simulink library "inp"  (R2021b)
settings: Solver=VariableStepAuto  StartTime=0.0  StopTime=10.0  RelTol=1e-3
undefined symbols (not defined in the file): C_TASK_5MS_S, FALSE, KINP_AcoreReadyToSlp_flg_ovrdflg, KINP_AcoreReadyToSlp_flg_ovrdval, KINP_AllowMovThd_OTA_enum_ovrdflg, KINP_AllowMovThd_OTA_enum_ovrdval, KINP_APSAngleTarget_Deg_ovrdflg, KINP_APSAngleTarget_Deg_ovrdval, KINP_APSDecReq_mps2_ovrdflg, KINP_APSDecReq_mps2_ovrdval, KINP_APSDecReqA_flg_ovrdflg, KINP_APSDecReqA_flg_ovrdval, KINP_APSDFLL_cm_ovrdflg, KINP_APSDFLL_cm_ovrdval, KINP_APSDFLR_cm_ovrdflg, KINP_APSDFLR_cm_ovrdval, KINP_APSDRLL_cm_ovrdflg, KINP_APSDRLL_cm_ovrdval, KINP_APSDRLR_cm_ovrdflg, KINP_APSDRLR_cm_ovrdval, KINP_APSExitCondition_enum_ovrdflg, KINP_APSExitCondition_enum_ovrdval, KINP_APSHWVer_enum_ovrdflg, KINP_APSHWVer_enum_ovrdval, KINP_APSProgressPCT_pct_ovrdflg, KINP_APSProgressPCT_pct_ovrdval, KINP_APSReq_enum_ovrdflg, KINP_APSReq_enum_ovrdval, KINP_APSRQDisplay_enum_ovrdflg, KINP_APSRQDisplay_enum_ovrdval, KINP_APSRqEPASCtrl_flg_ovrdflg, KINP_APSRqEPASCtrl_flg_ovrdval, KINP_APSShiftPosnReq_enum_ovrdval, KINP_APSShiftPosnReq_enum_ovrflg, KINP_APSSpeedCMD_kph_ovrdval, KINP_APSSpeedCMD_kph_ovrflg, KINP_APSStaSystem_enum_ovrdflg, KINP_APSStaSystem_enum_ovrdval, KINP_APSSWVer_enum_ovrdflg, KINP_APSSWVer_enum_ovrdval, KINP_APSVMCReqA_flg_ovrdval, KINP_APSVMCReqA_flg_ovrflg, KINP_APSVRqEPASCtrl_flg_ovrdflg, KINP_APSVRqEPASCtrl_flg_ovrdval, KINP_AuxBattVolmV_mV_ovrdflg, KINP_AuxBattVolmV_mV_ovrdval, KINP_CAASSta_enum_ovrdflg, KINP_CAASSta_enum_ovrdval, KINP_CAASVMCReqA_flg_ovrdval, KINP_CAASVMCReqA_flg_ovrflg, KINP_Chime_enum_ovrdflg, KINP_Chime_enum_ovrdval, KINP_ClearDTCcmd_flg_ovrdflg, KINP_ClearDTCcmd_flg_ovrdval, KINP_EvccAplusPwrUpReq_flg_ovrdflg, KINP_EvccAplusPwrUpReq_flg_ovrdval, KINP_LFID_raw_ovrdval, KINP_LFID_raw_ovrflg, KINP_LRID_raw_ovrdval, KINP_MemOffsetAccX_raw16_ovrdflg ... (+118)
libraries: FVT_lib x595, hcu_lib x1
(part 27 of 27)

== system inp/INP/CAN5/SignalCheck/TBOX1 ==
  BHAL_outputs : Inport
  inp_CanValid_bus : Inport  Port=2
  PowerOffTSet : FVT_lib/inp/can_signal_template  SystemSampleTime=-1  VariantActivationTime=update diagram  Latency=0  AutoFrameSizeCalculation=off
      link override defval: Value=KINP_PowerOffTSet_cnt_defval
      link override fftdec: Value=KINP_PowerOffTSet_cnt_fftdec
      link override fftinc: Value=KINP_PowerOffTSet_cnt_fftinc
      link override fftlim: Value=KINP_PowerOffTSet_cnt_fftlim
      link override invalid: Value=KINP_PowerOffTSet_cnt_invalid
      link override ovrdflg: Value=KINP_PowerOffTSet_cnt_ovrdflg
      link override ovrdval: Value=KINP_PowerOffTSet_cnt_ovrdval
      link override setvalid: Value=KINP_PowerOffTSet_cnt_setvalid
      link override srvcflg: Value=KINP_PowerOffTSet_cnt_srvcflg
      link override srvcval: Value=KINP_PowerOffTSet_cnt_srvcval
  ReDoorLock : FVT_lib/inp/can_signal_template  SystemSampleTime=-1  VariantActivationTime=update diagram  Latency=0  AutoFrameSizeCalculation=off
      link override defval: Value=KINP_ReDoorLock_enum_defval
      link override fftdec: Value=KINP_ReDoorLock_enum_fftdec
      link override fftinc: Value=KINP_ReDoorLock_enum_fftinc
      link override fftlim: Value=KINP_ReDoorLock_enum_fftlim
      link override invalid: Value=KINP_ReDoorLock_enum_invalid
      link override ovrdflg: Value=KINP_ReDoorLock_enum_ovrdflg
      link override ovrdval: Value=KINP_ReDoorLock_enum_ovrdval
      link override setvalid: Value=KINP_ReDoorLock_enum_setvalid
      link override srvcflg: Value=KINP_ReDoorLock_enum_srvcflg
      link override srvcval: Value=KINP_ReDoorLock_enum_srvcval
  ReOutsideMirror : FVT_lib/inp/can_signal_template  SystemSampleTime=-1  VariantActivationTime=update diagram  Latency=0  AutoFrameSizeCalculation=off
      link override defval: Value=KINP_ReOutsideMirror_enum_defval
      link override fftdec: Value=KINP_ReOutsideMirror_enum_fftdec
      link override fftinc: Value=KINP_ReOutsideMirror_enum_fftinc
      link override fftlim: Value=KINP_ReOutsideMirror_enum_fftlim
      link override invalid: Value=KINP_ReOutsideMirror_enum_invalid
      link override ovrdflg: Value=KINP_ReOutsideMirror_enum_ovrdflg
      link override ovrdval: Value=KINP_ReOutsideMirror_enum_ovrdval
      link override setvalid: Value=KINP_ReOutsideMirror_enum_setvalid
      link override srvcflg: Value=KINP_ReOutsideMirror_enum_srvcflg
      link override srvcval: Value=KINP_ReOutsideMirror_enum_srvcval
  RePwrReqTbox : FVT_lib/inp/can_signal_template  SystemSampleTime=-1  VariantActivationTime=update diagram  Latency=0  AutoFrameSizeCalculation=off
      link override defval: Value=KINP_RePwrReqTbox_enum_defval
      link override fftdec: Value=KINP_RePwrReqTbox_enum_fftdec
      link override fftinc: Value=KINP_RePwrReqTbox_enum_fftinc
      link override fftlim: Value=KINP_RePwrReqTbox_enum_fftlim
      link override invalid: Value=KINP_RePwrReqTbox_enum_invalid
      link override ovrdflg: Value=KINP_RePwrReqTbox_enum_ovrdflg
      link override ovrdval: Value=KINP_RePwrReqTbox_enum_ovrdval
      link override setvalid: Value=KINP_RePwrReqTbox_enum_setvalid
      link override srvcflg: Value=KINP_RePwrReqTbox_enum_srvcflg
      link override srvcval: Value=KINP_RePwrReqTbox_enum_srvcval
  RemoteACTemp : FVT_lib/inp/can_signal_template  SystemSampleTime=-1  VariantActivationTime=update diagram  Latency=0  AutoFrameSizeCalculation=off
      link override defval: Value=KINP_RemoteACTemp_C_defval
      link override fftdec: Value=KINP_RemoteACTemp_C_fftdec
      link override fftinc: Value=KINP_RemoteACTemp_C_fftinc
      link override fftlim: Value=KINP_RemoteACTemp_C_fftlim
      link override invalid: Value=KINP_RemoteACTemp_C_invalid
      link override ovrdflg: Value=KINP_RemoteACTemp_C_ovrdflg
      link override ovrdval: Value=KINP_RemoteACTemp_C_ovrdval
      link override setvalid: Value=KINP_RemoteACTemp_C_setvalid
      link override srvcflg: Value=KINP_RemoteACTemp_C_srvcflg
      link override srvcval: Value=KINP_RemoteACTemp_C_srvcval
  RemoteAutoReq : FVT_lib/inp/can_signal_template  SystemSampleTime=-1  VariantActivationTime=update diagram  Latency=0  AutoFrameSizeCalculation=off
      link override defval: Value=KINP_RemoteAutoReq_flg_defval
      link override fftdec: Value=KINP_RemoteAutoReq_flg_fftdec
      link override fftinc: Value=KINP_RemoteAutoReq_flg_fftinc
      link override fftlim: Value=KINP_RemoteAutoReq_flg_fftlim
      link override invalid: Value=KINP_RemoteAutoReq_flg_invalid
      link override ovrdflg: Value=KINP_RemoteAutoReq_flg_ovrdflg
      link override ovrdval: Value=KINP_RemoteAutoReq_flg_ovrdval
      link override setvalid: Value=KINP_RemoteAutoReq_flg_setvalid
      link override srvcflg: Value=KINP_RemoteAutoReq_flg_srvcflg
      link override srvcval: Value=KINP_RemoteAutoReq_flg_srvcval
  Terminator_{1..6} (6 alike) : Terminator
  True_VHAL_PowerOffTSet_cnt : Constant  Value=TRUE  OutDataTypeStr=boolean
  True_VHAL_ReDoorLock_enum : Constant  Value=TRUE  OutDataTypeStr=boolean
  True_VHAL_ReOutsideMirror_enum : Constant  Value=TRUE  OutDataTypeStr=boolean
  True_VHAL_RePwrReqTbox_enum : Constant  Value=TRUE  OutDataTypeStr=boolean
  True_VHAL_RemoteACTemp_C : Constant  Value=TRUE  OutDataTypeStr=boolean
  True_VHAL_RemoteAutoReq_flg : Constant  Value=TRUE  OutDataTypeStr=boolean
  slr1_{1..6} (6 alike) : BusSelector  OutputSignals=VINP_CANMsgValidTBOX1_flg
  slr_VHAL_PowerOffTSet_cnt : BusSelector  OutputSignals=VHAL_PowerOffTSet_cnt
  slr_VHAL_ReDoorLock_enum : BusSelector  OutputSignals=VHAL_ReDoorLock_enum
  slr_VHAL_ReOutsideMirror_enum : BusSelector  OutputSignals=VHAL_ReOutsideMirror_enum
  slr_VHAL_RePwrReqTbox_enum : BusSelector  OutputSignals=VHAL_RePwrReqTbox_enum
  slr_VHAL_RemoteACTemp_C : BusSelector  OutputSignals=VHAL_RemoteACTemp_C
  slr_VHAL_RemoteAutoReq_flg : BusSelector  OutputSignals=VHAL_RemoteAutoReq_flg
  VINP_PowerOffTSet_cnt : Outport
  VINP_ReOutsideMirror_enum : Outport  Port=2
  VINP_ReDoorLock_enum : Outport  Port=3
  VINP_RePwrReqTbox_enum : Outport  Port=4
  VINP_RemoteACTemp_C : Outport  Port=5
  VINP_RemoteAutoReq_flg : Outport  Port=6
  wires:
  BHAL_outputs/1 -> [BHAL_outputs]
  inp_CanValid_bus/1 -> [inp_CanValid_bus]
  [BHAL_outputs] -> slr_VHAL_PowerOffTSet_cnt/1
  slr_VHAL_PowerOffTSet_cnt/1 -> PowerOffTSet/1  "<VHAL_PowerOffTSet_cnt>"
  True_VHAL_PowerOffTSet_cnt/1 -> PowerOffTSet/2
  [inp_CanValid_bus] -> slr1_1/1
  slr1_1/1 -> PowerOffTSet/3  "<VINP_CANMsgValidTBOX1_flg>"
  PowerOffTSet/1 -> VINP_PowerOffTSet_cnt/1  "VINP_PowerOffTSet_cnt"
  PowerOffTSet/2 -> Terminator_1/1
  [BHAL_outputs] -> slr_VHAL_ReOutsideMirror_enum/1
  slr_VHAL_ReOutsideMirror_enum/1 -> ReOutsideMirror/1  "<VHAL_ReOutsideMirror_enum>"
  True_VHAL_ReOutsideMirror_enum/1 -> ReOutsideMirror/2
  [inp_CanValid_bus] -> slr1_2/1
  slr1_2/1 -> ReOutsideMirror/3  "<VINP_CANMsgValidTBOX1_flg>"
  ReOutsideMirror/1 -> VINP_ReOutsideMirror_enum/1  "VINP_ReOutsideMirror_enum"
  ReOutsideMirror/2 -> Terminator_2/1
  [BHAL_outputs] -> slr_VHAL_ReDoorLock_enum/1
  slr_VHAL_ReDoorLock_enum/1 -> ReDoorLock/1  "<VHAL_ReDoorLock_enum>"
  True_VHAL_ReDoorLock_enum/1 -> ReDoorLock/2
  [inp_CanValid_bus] -> slr1_3/1
  slr1_3/1 -> ReDoorLock/3  "<VINP_CANMsgValidTBOX1_flg>"
  ReDoorLock/1 -> VINP_ReDoorLock_enum/1  "VINP_ReDoorLock_enum"
  ReDoorLock/2 -> Terminator_3/1
  [BHAL_outputs] -> slr_VHAL_RePwrReqTbox_enum/1
  slr_VHAL_RePwrReqTbox_enum/1 -> RePwrReqTbox/1  "<VHAL_RePwrReqTbox_enum>"
  True_VHAL_RePwrReqTbox_enum/1 -> RePwrReqTbox/2
  [inp_CanValid_bus] -> slr1_4/1
  slr1_4/1 -> RePwrReqTbox/3  "<VINP_CANMsgValidTBOX1_flg>"
  RePwrReqTbox/1 -> VINP_RePwrReqTbox_enum/1  "VINP_RePwrReqTbox_enum"
  RePwrReqTbox/2 -> Terminator_4/1
  [BHAL_outputs] -> slr_VHAL_RemoteACTemp_C/1
  slr_VHAL_RemoteACTemp_C/1 -> RemoteACTemp/1  "<VHAL_RemoteACTemp_C>"
  True_VHAL_RemoteACTemp_C/1 -> RemoteACTemp/2
  [inp_CanValid_bus] -> slr1_5/1
  slr1_5/1 -> RemoteACTemp/3  "<VINP_CANMsgValidTBOX1_flg>"
  RemoteACTemp/1 -> VINP_RemoteACTemp_C/1  "VINP_RemoteACTemp_C"
  RemoteACTemp/2 -> Terminator_5/1
  [BHAL_outputs] -> slr_VHAL_RemoteAutoReq_flg/1
  slr_VHAL_RemoteAutoReq_flg/1 -> RemoteAutoReq/1  "<VHAL_RemoteAutoReq_flg>"
  True_VHAL_RemoteAutoReq_flg/1 -> RemoteAutoReq/2
  [inp_CanValid_bus] -> slr1_6/1
  slr1_6/1 -> RemoteAutoReq/3  "<VINP_CANMsgValidTBOX1_flg>"
  RemoteAutoReq/1 -> VINP_RemoteAutoReq_flg/1  "VINP_RemoteAutoReq_flg"
  RemoteAutoReq/2 -> Terminator_6/1
